simulink model "fig7_54"  (Simulink 7.9)
settings: Solver=ode23  StartTime=0.0  StopTime=5  RelTol=1e-3
settings Model: Creator=abbas  LastModifiedBy=abbas  ExtModeTrigMode=oneshot  ExtModeArmWhenConnect=off
settings DataIOCC: LimitDataPoints=off
settings OptimizationCC: BlockReduction=off  BooleanDataType=off  InlineInvariantSignals=on  InitFltsAndDblsToZero=on
settings DebuggingCC: SaveWithParameterizedLinksMsg=none  SignalResolutionControl=TryResolveAllWithWarning  SolverPrmCheckMsg=none  MultiTaskDSMMsg=warning  MultiTaskCondExecSysMsg=none  FcnCallInpInsideContextMsg=Use local settings  StrictBusMsg=None
settings HardwareCC: TargetUnknown=on
settings RTWCC: IncludeERTFirstTime=on
settings GRTTargetCC: TargetFcnLib=ansi_tfl_tmw.mat  ModelReferenceCompliant=off  ParMdlRefBuildCompliant=off  CompOptLevelCompliant=off  ConcurrentExecutionCompliant=off  CombineOutputUpdateFcns=off  MatFileLogging=off  GRTInterface=on

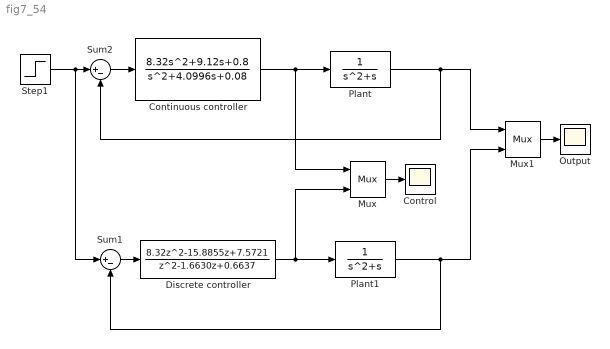
== system fig7_54 ==
  Continuous controller : TransferFcn  Numerator=[8.32 9.12 0.8]  Denominator=[1 4.0996 0.08]
  Control : Scope
      settings: TickLabels=on  YMin=0  YMax=2.75  SaveName=ucd
  Discrete controller : DiscreteTransferFcn  Numerator="[8.32  -15.8855 7.5721]"  Denominator=[1 -1.6630 0.6637]  SampleTime=.1
  Mux : Mux  Inputs=2
  Mux1 : Mux  Inputs=2
  Output : Scope
      settings: TickLabels=on  YMin=1.0035  YMax=1.01  SaveName=ycd
  Plant : TransferFcn  Denominator="[1  1 0]"
  Plant1 : TransferFcn  Denominator="[1  1 0]"
  Step1 : Step  Time=0  SampleTime=.001
  Sum1 : Sum  Inputs=|+-  InputSameDT=on  OutDataTypeStr=Inherit: Same as first input
  Sum2 : Sum  Inputs=|+-  InputSameDT=on  OutDataTypeStr=Inherit: Same as first input
  wires:
  Step1/1 -> Sum2/1, Sum1/1
  Mux/1 -> Control/1
  Mux1/1 -> Output/1
  Sum1/1 -> Discrete controller/1
  Plant1/1 -> Mux1/2, Sum1/2
  Plant/1 -> Mux1/1, Sum2/2
  Sum2/1 -> Continuous controller/1
  Continuous controller/1 -> Mux/1, Plant/1
  Discrete controller/1 -> Mux/2, Plant1/1
